simulink model "chap7_1sim"  (Simulink 8.3)
settings: Solver=ode45  StartTime=0.0  StopTime=10.0  RelTol=1e-3
settings Model: Creator=Ntlldn  LastModifiedBy=Administrator
settings SolverCC: ZeroCrossControl=DisableAll
settings DataIOCC: LimitDataPoints=off  SignalLoggingSaveFormat=Dataset
settings OptimizationCC: LifeSpan=auto
settings DebuggingCC: UnderspecifiedInitializationDetection=Simplified  MergeDetectMultiDrivingBlocksExec=error  SolverPrmCheckMsg=none  FrameProcessingCompatibilityMsg=error  StateNameClashWarn=none  SFUnexpectedBacktrackingDiag=error  SFNoUnconditionalDefaultTransitionDiag=error
settings HardwareCC: ProdBitPerPointer=64  ProdLargestAtomicFloat=Float  ProdIntDivRoundTo=Zero  ProdEndianess=LittleEndian  ProdWordSize=64  ProdLongLongMode=on  ProdHWDeviceType=Intel->x86-64 (Windows64)
settings ModelReferenceCC: PropagateSignalLabelsOutOfModel=on
settings SFSimCC: SimUseLocalCustomCode=on
settings RTWCC: RTWUseLocalCustomCode=on
settings GRTTargetCC: TargetLangStandard=C99 (ISO)  GeneratePreprocessorConditionals=Use local settings  CombineOutputUpdateFcns=on  GRTInterface=off

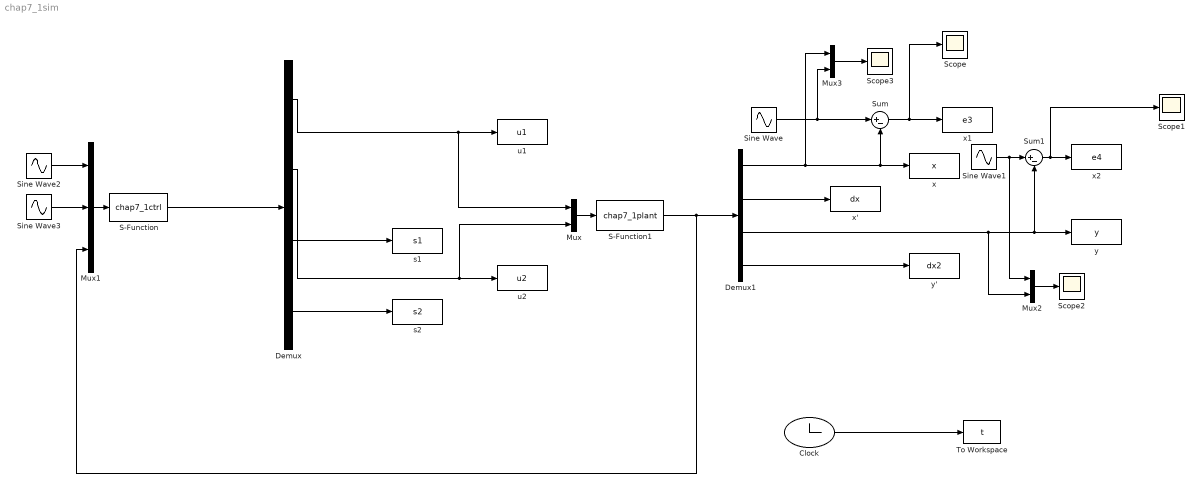
== system chap7_1sim ==
  Clock : Clock
  Demux : Demux
  Demux1 : Demux
  Mux : Mux  Inputs=2
  Mux1 : Mux  Inputs=3
  Mux2 : Mux  Inputs=2
  Mux3 : Mux  Inputs=2
  S-Function : S-Function  FunctionName=chap7_1ctrl  EnableBusSupport=off
  S-Function1 : S-Function  FunctionName=chap7_1plant  EnableBusSupport=off
  Scope{,1..3} (4 alike) : Scope
  Sine Wave : Sin  Frequency=4.17  SampleTime=0
  Sine Wave1 : Sin  Amplitude=0.7  Frequency=5.67  SampleTime=0
  Sine Wave2 : Sin  Frequency=4.17  SampleTime=0
  Sine Wave3 : Sin  Amplitude=0.7  Frequency=5.67  SampleTime=0
  Sum : Sum  Inputs=|+-
  Sum1 : Sum  Inputs=|+-
  To Workspace : ToWorkspace  VariableName=t  SampleTime=-1
  s1 : ToWorkspace  VariableName=s1  SampleTime=-1
  s2 : ToWorkspace  VariableName=s2  SampleTime=-1
  u1 : ToWorkspace  VariableName=u1  SampleTime=-1
  u2 : ToWorkspace  VariableName=u2  SampleTime=-1
  x : ToWorkspace  VariableName=x  SampleTime=-1
  x' : ToWorkspace  VariableName=dx  SampleTime=-1
  x1 : ToWorkspace  VariableName=e3  SampleTime=-1
  x2 : ToWorkspace  VariableName=e4  SampleTime=-1
  y : ToWorkspace  VariableName=y  SampleTime=-1
  y' : ToWorkspace  VariableName=dx2  SampleTime=-1
  wires:
  Demux/2 -> u2/1, Mux/2
  Sum1/1 -> x2/1, Scope1/1
  Mux/1 -> S-Function1/1
  Sine Wave1/1 -> Sum1/1, Mux2/1
  Demux1/1 -> x/1, Sum/2, Mux3/1
  S-Function1/1 -> Demux1/1, Mux1/3
  Mux2/1 -> Scope2/1
  S-Function/1 -> Demux/1
  Demux/1 -> Mux/1, u1/1
  Sine Wave3/1 -> Mux1/2
  Demux1/3 -> y/1, Sum1/2, Mux2/2
  Demux1/2 -> x'/1
  Mux1/1 -> S-Function/1
  Sine Wave2/1 -> Mux1/1
  Sine Wave/1 -> Sum/1, Mux3/2
  Sum/1 -> x1/1, Scope/1
  Clock/1 -> To Workspace/1
  Demux1/4 -> y'/1
  Mux3/1 -> Scope3/1
  Demux/3 -> s1/1
  Demux/4 -> s2/1
